simulink model "IMC_grau_relativo_1_20140204"  (Simulink 7.9)
settings: Solver=ode45  StartTime=0.0  StopTime=5  FixedStep=Ts  RelTol=1e-3
InitFcn:
  | IMC_ini
values from neighbouring files (symbols this model uses):
  Ts = 0.5    [IMC_calculo_limites_thetas.m]    (also in IMC_datta_ini.m; IMC_ini.m = 8.33333333333e-05; JORGE_controlador_LCL_malha_interna.m = 8.33333333333e-05; LCL_PAPM.m = 8.33333333333e-05)
undefined symbols (not defined in the file or in its folder): PD, PN
settings Model: Creator=Marcelo  LastModifiedBy=marcelodurgante
settings SolverCC: AutoInsertRateTranBlk=on
settings OptimizationCC: ExpressionDepthLimit=128
settings CodeAppCC: CustomSymbolStrType=$N$R$M_T
settings GRTTargetCC: CombineOutputUpdateFcns=off  GRTInterface=on

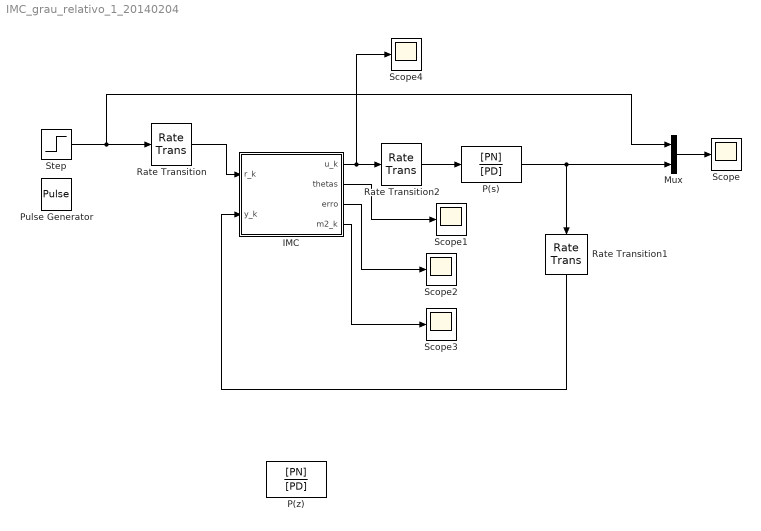
== system IMC_grau_relativo_1_20140204 ==
  IMC : MATLAB Function  TreatAsAtomicUnit=on
  Mux : Mux  Inputs=2
  P(s) : TransferFcn  Numerator=[PN]  Denominator=[PD]
  P(z) : DiscreteTransferFcn  Numerator=[PN]  Denominator=[PD]  SampleTime=Ts
  Pulse Generator : DiscretePulseGenerator  PulseType=Time based  PulseWidth=50
  Rate Transition : RateTransition  OutPortSampleTime=Ts
  Rate Transition1 : RateTransition  OutPortSampleTime=Ts
  Rate Transition2 : RateTransition  OutPortSampleTime=Ts
  Scope{,1..4} (5 alike) : Scope
      Scope settings: TimeRange=0.002313752565402893  YMin=0.0006465729097369394  YMax=0.0006738845294319801
      Scope2 settings: SaveName=ScopeData2
      Scope3 settings: SaveName=ScopeData3
      Scope4 settings: SaveName=ScopeData4
  Step : Step  Before=0.5  After=1.5  SampleTime=0
  wires:
  P(s)/1 -> Rate Transition1/1, Mux/2
  Mux/1 -> Scope/1
  Rate Transition2/1 -> P(s)/1
  IMC/1(u_k) -> Rate Transition2/1, Scope4/1
  Rate Transition/1 -> IMC/1(r_k)
  Rate Transition1/1 -> IMC/2(y_k)
  IMC/2(thetas) -> Scope1/1
  IMC/3(erro) -> Scope2/1
  IMC/4(m2_k) -> Scope3/1
  Step/1 -> Rate Transition/1, Mux/1

== matlab function IMC ==
  data: r_k input double; y_k input double; u_k output double; thetas output double; erro output double; m2_k output double
function [u_k, thetas, erro, m2_k] = imc(r_k, y_k)
%#CODEGEN

%ganho adaptativo entre 0 e 0.5
gamma=0.45;

%constante escolhida entre 0 e 1
delta0=0.99;

%lambdas escolhidos de forma que Lambda seja estável - coeficientes de (z-0.1)^3
lambda0=-0.001;
lambda1= 0.03;
lambda2=-0.3;

%definição do conjunto no qual serão projetados os parâmetros
%thetas estrela

theta_e=[-1.0537; 0.7138; 0.9190; 0.0166; 0.0423; 0.0160];
min=0.1;
max=10;
theta1_min=theta_e(1)*min;
theta1_max=theta_e(1)*max;
theta2_min=theta_e(2)*min;
theta2_max=theta_e(2)*max;
theta3_min=theta_e(3)*min;
theta3_max=theta_e(3)*max;
theta4_min=theta_e(4)*min;
theta4_max=theta_e(4)*max;
theta5_min=theta_e(5)*min;
theta5_max=theta_e(5)*max;
theta6_min=theta_e(6)*min;
theta6_max=theta_e(6)*max;


%% Declarações

persistent theta_k;
if isempty(theta_k)
    theta_k=[min*theta_e(1); min*theta_e(2); max*theta_e(3); min*theta_e(4); max*theta_e(5); max*theta_e(6)];
end

persistent phi11_k1;
if isempty(phi11_k1)
    phi11_k1=0;
end

persistent phi11_k2;
if isempty(phi11_k2)
    phi11_k2=0;
end

persistent phi11_k3;
if isempty(phi11_k3)
    phi11_k3=0;
end

persistent phi12_k1;
if isempty(phi12_k1)
    phi12_k1=0;
end

persistent phi12_k2;
if isempty(phi12_k2)
    phi12_k2=0;
end

persistent phi12_k3;
if isempty(phi12_k3)
    phi12_k3=0;
end

persistent phi13_k1;
if isempty(phi13_k1)
    phi13_k1=0;
end

persistent phi13_k2;
if isempty(phi13_k2)
    phi13_k2=0;
end

persistent phi13_k3;
if isempty(phi13_k3)
    phi13_k3=0;
end

persistent phi21_k1;
if isempty(phi21_k1)
    phi21_k1=0;
end

persistent phi21_k2;
if isempty(phi21_k2)
    phi21_k2=0;
end

persistent phi21_k3;
if isempty(phi21_k3)
    phi21_k3=0;
end

persistent phi22_k1;
if isempty(phi22_k1)
    phi22_k1=0;
end

persistent phi22_k2;
if isempty(phi22_k2)
    phi22_k2=0;
end

persistent phi22_k3;
if isempty(phi22_k3)
    phi22_k3=0;
end

persistent phi23_k1;
if isempty(phi23_k1)
    phi23_k1=0;
end

persistent phi23_k2;
if isempty(phi23_k2)
    phi23_k2=0;
end

persistent phi23_k3;
if isempty(phi23_k3)
    phi23_k3=0;
end

persistent u_k1;
if isempty(u_k1)
    u_k1=0;
end

persistent u_k2;
if isempty(u_k2)
    u_k2=0;
end

persistent u_k3;
if isempty(u_k3)
    u_k3=0;
end

persistent y_k1;
if isempty(y_k1)
    y_k1=0;
end

persistent y_k2;
if isempty(y_k2)
    y_k2=0;
end

persistent y_k3;
if isempty(y_k3)
    y_k3=0;
end

persistent rer_k1;
if isempty(rer_k1)
    rer_k1=0;
end

persistent rer_k2;
if isempty(rer_k2)
    rer_k2=0;
end

persistent rer_k3;
if isempty(rer_k3)
    rer_k3=0;
end

persistent m2;
if isempty(m2)
    m2=1;
end

%% Cálculos

phi11_k = y_k1 - lambda2*phi11_k1 - lambda1*phi11_k2 - lambda0*phi11_k3;
phi12_k = y_k2 - lambda2*phi12_k1 - lambda1*phi12_k2 - lambda0*phi12_k3;
phi13_k = y_k3 - lambda2*phi13_k1 - lambda1*phi13_k2 - lambda0*phi13_k3;
phi21_k = u_k1 - lambda2*phi21_k1 - lambda1*phi21_k2 - lambda0*phi21_k3;
phi22_k = u_k2 - lambda2*phi22_k1 - lambda1*phi22_k2 - lambda0*phi22_k3;
phi23_k = u_k3 - lambda2*phi23_k1 - lambda1*phi23_k2 - lambda0*phi23_k3;

phi1_k=[phi11_k phi12_k phi13_k];
phi2_k=[phi21_k phi22_k phi23_k];

phi_k = [phi1_k'; phi2_k'];

m2_k= m2 + phi_k'*phi_k;

y_hat_k= theta_k'*phi_k;

eta_k= (y_k - y_hat_k)/m2_k;

erro = eta_k;

%Elementos auxiliares no cálculo da ação de controle
%delta_b=real(sqrt(complex(theta_k(5)^2-4*theta_k(4)*theta_k(6))));
delta_b=sqrt(theta_k(5)^2-4*theta_k(4)*theta_k(6));
phi=2*theta_k(4)/(-theta_k(5)-delta_b);
z_fm=(-theta_k(5)+delta_b)/(2*theta_k(4));
%z_fm=phi;
rer_k= r_k - (y_k - y_hat_k);

%Ganho para Q com pólos contendo parte real negativa
%G=(1-phi)/(1-(1/phi));
%Ganho para Q sem pólos com parte real negativa
G=((1-phi)/(1-(1/phi)))*(1/((1-phi)*(1-z_fm)));

%Cálculo da ação de controle (deixando os pólos com parte real negativa)
%u_k= G*(rer_k + (lambda2-theta_k(1))*rer_k1 + (lambda1-theta_k(2))*rer_k2 + (lambda0-theta_k(3))*rer_k3) ...
%    + (phi+z_fm)*u_k1 - phi*z_fm*u_k2;

%Cálculo da ação de controle (retirando os pólos com parte real negativa
%via Q_c - ver no artigo do Datta)
u_k= G*(rer_k + (lambda2-theta_k(1))*rer_k1 + (lambda1-theta_k(2))*rer_k2 + (lambda0-theta_k(3))*rer_k3);


%% Atualização

m2 = delta0*(m2 - 1) + u_k^2 + y_k^2 + 1;

%atualização de theta_k via algoritmo de projeção de parâmetros
g1_k= -gamma*eta_k*phi11_k;
g2_k= -gamma*eta_k*phi12_k;
g3_k= -gamma*eta_k*phi13_k;
g4_k= -gamma*eta_k*phi21_k;
g5_k= -gamma*eta_k*phi22_k;
g6_k= -gamma*eta_k*phi23_k;

f1_k=0;
if (theta_k(1)+g1_k)>theta1_max
    f1_k=theta1_max-theta_k(1)-g1_k;
end
if (theta_k(1)+g1_k)<theta1_min
    f1_k=theta1_min-theta_k(1)-g1_k;
end

f2_k=0;
if (theta_k(2)+g2_k)>theta2_max
    f2_k=theta2_max-theta_k(2)-g2_k;
end
if (theta_k(2)+g2_k)<theta2_min
    f2_k=theta2_min-theta_k(2)-g2_k;
end

f3_k=0;
if (theta_k(3)+g3_k)>theta3_max
    f3_k=theta3_max-theta_k(3)-g3_k;
end
if (theta_k(3)+g3_k)<theta3_min
    f3_k=theta3_min-theta_k(3)-g3_k;
end

f4_k=0;
if (theta_k(4)+g4_k)>theta4_max
    f4_k=theta4_max-theta_k(4)-g4_k;
end
if (theta_k(4)+g4_k)<theta4_min
    f4_k=theta4_min-theta_k(4)-g4_k;
end

f5_k=0;
if (theta_k(5)+g5_k)>theta5_max
    f5_k=theta5_max-theta_k(5)-g5_k;
end
if (theta_k(5)+g5_k)<theta5_min
    f5_k=theta5_min-theta_k(5)-g5_k;
end

f6_k=0;
if (theta_k(6)+g6_k)>theta6_max
    f6_k=theta6_max-theta_k(6)-g6_k;
end
if (theta_k(6)+g6_k)<theta6_min
    f6_k=theta6_min-theta_k(6)-g6_k;
end

f_k = [f1_k; f2_k; f3_k; f4_k; f5_k; f6_k];

%theta_k = theta_k + gamma*eta_k*phi_k + f_k;

thetas = theta_k;


%atualização de estados anteriores
phi11_k3 = phi11_k2;
phi11_k2 = phi11_k1;
phi11_k1 = phi11_k;
phi12_k3 = phi12_k2;
phi12_k2 = phi12_k1;
phi12_k1 = phi12_k;
phi13_k3 = phi13_k2;
phi13_k2 = phi13_k1;
phi13_k1 = phi13_k;
phi21_k3 = phi21_k2;
phi21_k2 = phi21_k1;
phi21_k1 = phi21_k;
phi22_k3 = phi22_k2;
phi22_k2 = phi22_k1;
phi22_k1 = phi22_k;
phi23_k3 = phi23_k2;
phi23_k2 = phi23_k1;
phi23_k1 = phi23_k;

u_k3 = u_k2;
u_k2 = u_k1;
u_k1 = u_k;

y_k3 = y_k2;
y_k2 = y_k1;
y_k1 = y_k;

rer_k3 = rer_k2;
rer_k2 = rer_k1;
rer_k1 = rer_k;


end
